simulink model "echo_ref"  (R2020b)
settings: Solver=FixedStepDiscrete  StartTime=0.0  StopTime=stopTime  RelTol=1e-3
undefined symbols (not defined in the file or in its folder): delay_dpram_addr_size
libraries: hdlsllib x4
settings Model: Creator=Ross  LastModifiedBy=wickh
settings SolverCC: MinimalZcImpactIntegration=on
settings DataIOCC: SaveOutput=off  SaveTime=off  ReturnWorkspaceOutputs=off
settings OptimizationCC: DefaultParameterBehavior=Inlined
settings DebuggingCC: ReadBeforeWriteMsg=DisableAll  WriteAfterWriteMsg=DisableAll  WriteAfterReadMsg=DisableAll  AlgebraicLoopMsg=error  MultiTaskDSMMsg=none  SingleTaskRateTransMsg=error  PregeneratedLibrarySubsystemCodeDiagnostic=none  ArithmeticOperatorsInVariantConditions=warning
settings HardwareCC: ProdBitPerPointer=32  ProdBitPerSizeT=32  ProdBitPerPtrDiffT=32  ProdLargestAtomicFloat=None  ProdIntDivRoundTo=Undefined  ProdEndianess=Unspecified  ProdWordSize=32  ProdHWDeviceType=ASIC/FPGA->ASIC/FPGA  TargetBitPerPointer=64  TargetBitPerSizeT=64  TargetBitPerPtrDiffT=64  TargetLongLongMode=on  TargetIntDivRoundTo=Zero  TargetEndianess=LittleEndian  TargetWordSize=64  TargetHWDeviceType=Custom Processor->MATLAB Host Computer  ProdEqTarget=off
settings ModelReferenceCC: UpdateModelReferenceTargets=IfOutOfDate
settings SFSimCC: SFSimEcho=off  SimUseLocalCustomCode=off  CustomCodeUndefinedFunction=UseInterfaceOnly
settings RTWCC: RTWUseLocalCustomCode=off

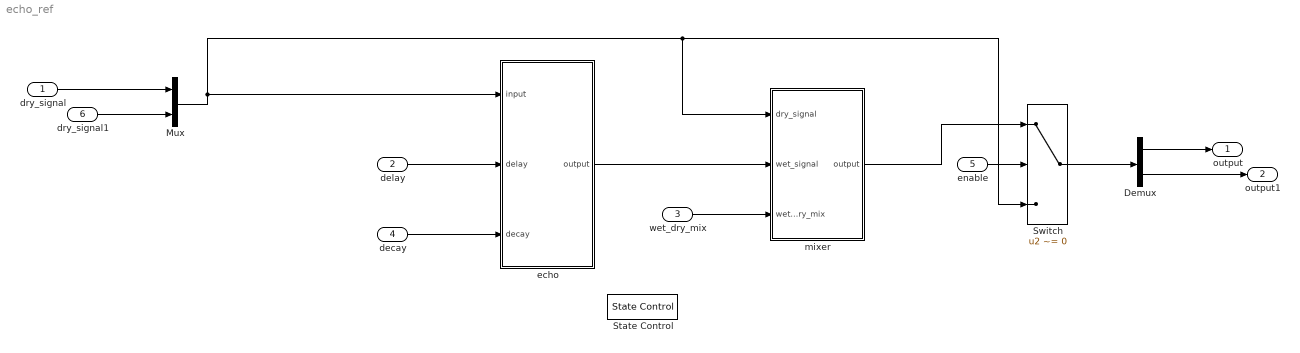
== system echo_ref ==
  dry_signal : Inport  OutDataTypeStr=mp.audio_dt  PortDimensions=1
  delay : Inport  Port=2  OutDataTypeStr=fixdt(0,15,0)  PortDimensions=1
  wet_dry_mix : Inport  Port=3  PortDimensions=1
  decay : Inport  Port=4  PortDimensions=1
  enable : Inport  Port=5  OutDataTypeStr=boolean
  dry_signal1 : Inport  Port=6  OutDataTypeStr=mp.audio_dt  PortDimensions=1
  Demux : Demux  Outputs=2
  Mux : Mux  Inputs=2
  State Control : StateControl  StateControl=Synchronous
  Switch : Switch  Criteria=u2 ~= 0
  echo : Subsystem
  mixer : Subsystem
  output : Outport  OutDataTypeStr=fixdt(1,24,23)  PortDimensions=1
  output1 : Outport  Port=2  OutDataTypeStr=fixdt(1,24,23)  PortDimensions=1
  wires:
  Mux/1 -> mixer/1(dry_signal), Switch/3, echo/1(input)
  echo/1(output) -> mixer/2(wet_signal)
  wet_dry_mix/1 -> mixer/3(wet_dry_mix)
  delay/1 -> echo/2(delay)
  mixer/1(output) -> Switch/1
  decay/1 -> echo/3(decay)
  enable/1 -> Switch/2
  dry_signal/1 -> Mux/1
  dry_signal1/1 -> Mux/2
  Switch/1 -> Demux/1
  Demux/1 -> output/1
  Demux/2 -> output1/1

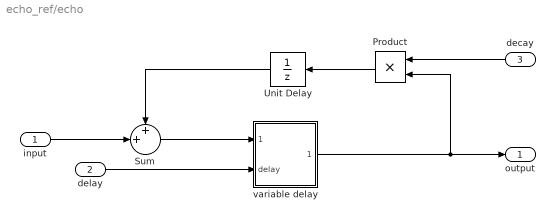
== system echo_ref/echo ==
  input : Inport
  delay : Inport  Port=2
  decay : Inport  Port=3  OutDataTypeStr=decay_dt
  Product : Product  OutDataTypeStr=fixdt(1,mp.W_bits,mp.F_bits)
  Sum : Sum  Inputs=++|
  Unit Delay : UnitDelay  SampleTime=-1  HasFrameUpgradeWarning=on
  variable delay : Subsystem
  output : Outport  VectorParamsAs1DForOutWhenUnconnected=off
  wires:
  decay/1 -> Product/1
  variable delay/1(data_out) -> Product/2, output/1
  Product/1 -> Unit Delay/1
  Unit Delay/1 -> Sum/1
  Sum/1 -> variable delay/1(data_in)
  input/1 -> Sum/2
  delay/1 -> variable delay/2(delay)

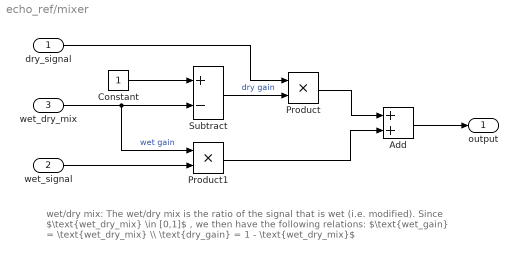
== system echo_ref/mixer ==
  note: wet/dry mix:
      | The wet/dry mix is the ratio of the signal that is wet (i.e. modified).
      |
      | Since $\text{wet_dry_mix} \in [0,1]$ , we then have the following relations:
      | $\text{wet_gain} = \text{wet_dry_mix} \\ \text{dry_gain} = 1 - \text{wet_dry_mix}$
  dry_signal : Inport
  wet_signal : Inport  Port=2
  wet_dry_mix : Inport  Port=3
  Add : Sum  OutDataTypeStr=fixdt(1,mp.W_bits,mp.F_bits)
  Constant : Constant  OutDataTypeStr=wet_dry_mix_dt  SampleTime=-1
  Product : Product
  Product1 : Product
  Subtract : Sum  Inputs=+-  InputSameDT=on  OutDataTypeStr=Inherit: Same as first input
  output : Outport  VectorParamsAs1DForOutWhenUnconnected=off
  wires:
  Constant/1 -> Subtract/1
  Add/1 -> output/1
  dry_signal/1 -> Product/1
  Subtract/1 -> Product/2  "dry gain"
  Product1/1 -> Add/2
  wet_signal/1 -> Product1/2
  Product/1 -> Add/1
  wet_dry_mix/1 -> Subtract/2, Product1/1  "wet gain"

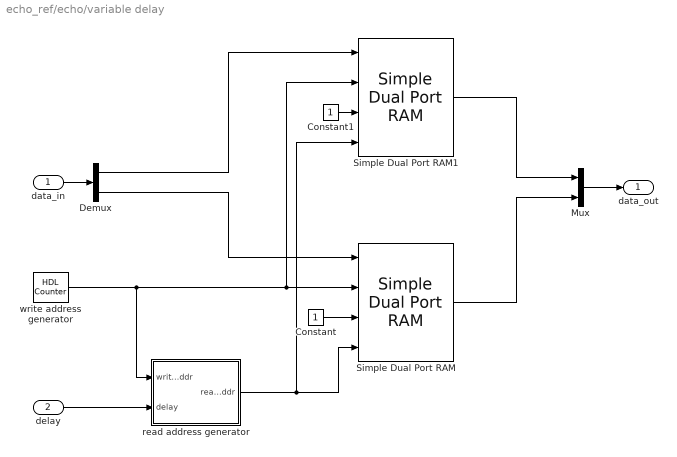
== system echo_ref/echo/variable delay ==
  data_in : Inport
  delay : Inport  Port=2
  Constant : Constant  OutDataTypeStr=Inherit: Inherit via back propagation  SampleTime=-1
  Constant1 : Constant  OutDataTypeStr=Inherit: Inherit via back propagation  SampleTime=-1
  Demux : Demux  Outputs=2
  Mux : Mux  Inputs=2
  Simple Dual Port RAM : hdlsllib/HDL RAMs/Simple Dual Port RAM  ram_size=delay_dpram_addr_size
      settings: SourceProductBaseCode=SL
  Simple Dual Port RAM1 : hdlsllib/HDL RAMs/Simple Dual Port RAM  ram_size=delay_dpram_addr_size
      settings: SourceProductBaseCode=SL
  read address generator : Subsystem
  write address generator : hdlsllib/Sources/HDL Counter  CountType=Count limited  CountInit=0  CountStep=1  CountMax=2^delay_dpram_addr_size - 1  CountFromType=Initial value  CountFrom=0  CountResetPort=off  CountLoadPort=off  CountEnbPort=off  CountDirPort=off  CountDataType=Unsigned  CountWordLen=delay_dpram_addr_size  CountFracLen=0  CountSampTime=-1
  data_out : Outport  VectorParamsAs1DForOutWhenUnconnected=off
  wires:
  Simple Dual Port RAM/1 -> Mux/2
  Simple Dual Port RAM1/1 -> Mux/1
  Mux/1 -> data_out/1
  Constant1/1 -> Simple Dual Port RAM1/3
  Demux/2 -> Simple Dual Port RAM/1
  Demux/1 -> Simple Dual Port RAM1/1
  data_in/1 -> Demux/1
  delay/1 -> read address generator/2(delay)
  read address generator/1(read_addr) -> Simple Dual Port RAM/4, Simple Dual Port RAM1/4
  write address generator/1 -> read address generator/1(write_addr), Simple Dual Port RAM/2, Simple Dual Port RAM1/2
  Constant/1 -> Simple Dual Port RAM/3

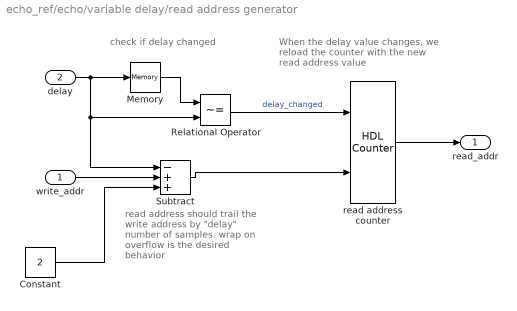
== system echo_ref/echo/variable delay/read address generator ==
  note: check if delay changed
  note: When the delay value changes, we reload the counter with the new read address value
  note: read address should trail the write address by "delay" number of samples.
      |
      | wrap on overflow is the desired behavior
  write_addr : Inport
  delay : Inport  Port=2
  Constant : Constant  Value=2  OutDataTypeStr=Inherit: Inherit via back propagation  SampleTime=-1
  Memory : Memory  InheritSampleTime=on
  Relational Operator : RelationalOperator  Operator=~=  OutDataTypeStr=boolean  RndMeth=Nearest
  Subtract : Sum  Inputs=-++  InputSameDT=on  OutDataTypeStr=Inherit: Same as first input
  read address counter : hdlsllib/Sources/HDL Counter  CountType=Count limited  CountInit=0  CountStep=1  CountMax=2^delay_dpram_addr_size - 1  CountFromType=Initial value  CountFrom=0  CountResetPort=off  CountLoadPort=on  CountEnbPort=off  CountDirPort=off  CountDataType=Unsigned  CountWordLen=delay_dpram_addr_size  CountFracLen=0  CountSampTime=-1
  read_addr : Outport  VectorParamsAs1DForOutWhenUnconnected=off
  wires:
  Constant/1 -> Subtract/3
  Subtract/1 -> read address counter/2
  write_addr/1 -> Subtract/2
  Relational Operator/1 -> read address counter/1  "delay_changed"
  Memory/1 -> Relational Operator/1
  delay/1 -> Subtract/1, Relational Operator/2, Memory/1
  read address counter/1 -> read_addr/1
